simulink model "Trab1_desafio_4"  (R2018a)
settings: Solver=VariableStepAuto  StartTime=0.0  StopTime=10.0  RelTol=1e-3
values from neighbouring files (symbols this model uses):
  A11 = Ad(1:k,1:k)    [Trab1_desafio4.m]
  A12 = Ad(1:k,k+1:end)    [Trab1_desafio4.m]
  A22 = Ad(k+1:end,k+1:end)    [Trab1_desafio4.m]
  B1 = Bd(1:k,:)    [Trab1_desafio4.m]
  C2 = Cd(:,k+1:end)    [Trab1_desafio4.m]
  z0_obs = z0(k+1:end,1)    [Trab1_desafio4.m]
  z0_uno = z0(1:k,1)    [Trab1_desafio4.m]
settings Model: Creator=eric-  LastModifiedBy=eric-

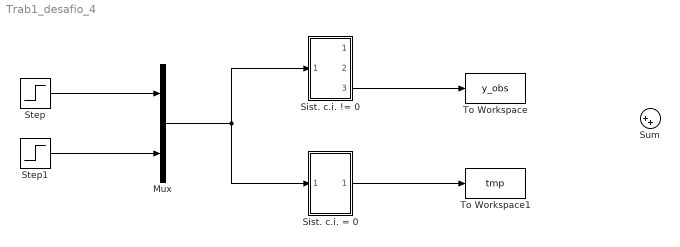
== system Trab1_desafio_4 ==
  Mux : Mux  Inputs=2
  Sist. c.i. != 0 : Subsystem
  Sist. c.i. = 0 : Subsystem
  Step : Step  SampleTime=0
  Step1 : Step  SampleTime=0
  Sum : Sum  Inputs=|++
  To Workspace : ToWorkspace  VariableName=y_obs  SaveFormat=Structure With Time  SampleTime=-1
  To Workspace1 : ToWorkspace  VariableName=tmp  SaveFormat=Structure With Time  SampleTime=-1
  wires:
  Step1/1 -> Mux/2
  Step/1 -> Mux/1
  Mux/1 -> Sist. c.i. != 0/1(In1), Sist. c.i. = 0/1(In1)
  Sist. c.i. = 0/1(Out1) -> To Workspace1/1
  Sist. c.i. != 0/3(Out3) -> To Workspace/1

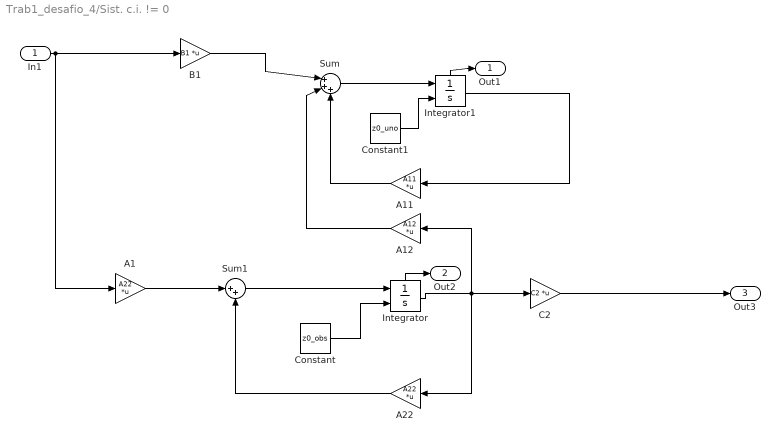
== system Trab1_desafio_4/Sist. c.i. != 0 ==
  In1 : Inport
  A1 : Gain  Gain=A22  Multiplication=Matrix(K*u)
  A11 : Gain  Gain=A11  Multiplication=Matrix(K*u)
  A12 : Gain  Gain=A12  Multiplication=Matrix(K*u)
  A22 : Gain  Gain=A22  Multiplication=Matrix(K*u)
  B1 : Gain  Gain=B1  Multiplication=Matrix(K*u)
  C2 : Gain  Gain=C2  Multiplication=Matrix(K*u)
  Constant : Constant  Value=z0_obs
  Constant1 : Constant  Value=z0_uno
  Integrator : Integrator  InitialConditionSource=external  ShowStatePort=on
  Integrator1 : Integrator  InitialConditionSource=external  ShowStatePort=on
  Sum : Sum  Inputs=|+++
  Sum1 : Sum  Inputs=|++
  Out1 : Outport
  Out2 : Outport  Port=2
  Out3 : Outport  Port=3
  wires:
  A1/1 -> Sum1/1
  Integrator1/1 -> A11/1
  Sum1/1 -> Integrator/1
  Integrator/1 -> A12/1, C2/1, A22/1
  B1/1 -> Sum/1
  Sum/1 -> Integrator1/1
  A22/1 -> Sum1/2
  Constant1/1 -> Integrator1/2
  A11/1 -> Sum/3
  Integrator1/State -> Out1/1
  Constant/1 -> Integrator/2
  A12/1 -> Sum/2
  C2/1 -> Out3/1
  Integrator/State -> Out2/1
  In1/1 -> A1/1, B1/1

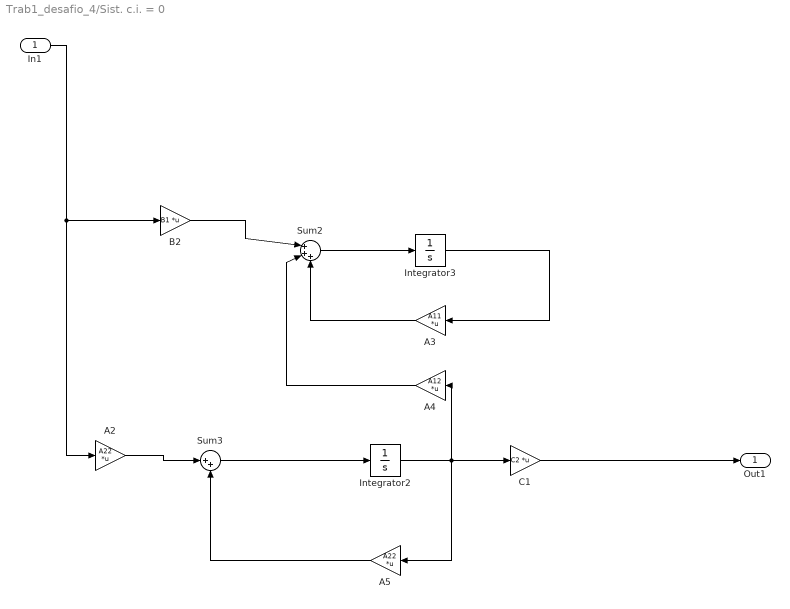
== system Trab1_desafio_4/Sist. c.i. = 0 ==
  In1 : Inport
  A2 : Gain  Gain=A22  Multiplication=Matrix(K*u)
  A3 : Gain  Gain=A11  Multiplication=Matrix(K*u)
  A4 : Gain  Gain=A12  Multiplication=Matrix(K*u)
  A5 : Gain  Gain=A22  Multiplication=Matrix(K*u)
  B2 : Gain  Gain=B1  Multiplication=Matrix(K*u)
  C1 : Gain  Gain=C2  Multiplication=Matrix(K*u)
  Integrator2 : Integrator
  Integrator3 : Integrator
  Sum2 : Sum  Inputs=|+++
  Sum3 : Sum  Inputs=|++
  Out1 : Outport
  wires:
  B2/1 -> Sum2/1
  A2/1 -> Sum3/1
  A5/1 -> Sum3/2
  A3/1 -> Sum2/3
  In1/1 -> A2/1, B2/1
  Integrator2/1 -> C1/1, A5/1, A4/1
  A4/1 -> Sum2/2
  Sum2/1 -> Integrator3/1
  Sum3/1 -> Integrator2/1
  C1/1 -> Out1/1
  Integrator3/1 -> A3/1
